simulink model "EV"  (R2022b)
settings: Solver=VariableStepAuto  StartTime=0.0  StopTime=500  RelTol=1e-3
libraries: autolibshared x1, slpidlib x1
settings Model: Creator=frz  LastModifiedBy=frz
settings SolverCC: ZeroCrossAlgorithm=Adaptive
settings DataIOCC: SaveOutput=off  SaveTime=off  ReturnWorkspaceOutputs=off
settings DebuggingCC: IgnoredZcDiagnostic=none

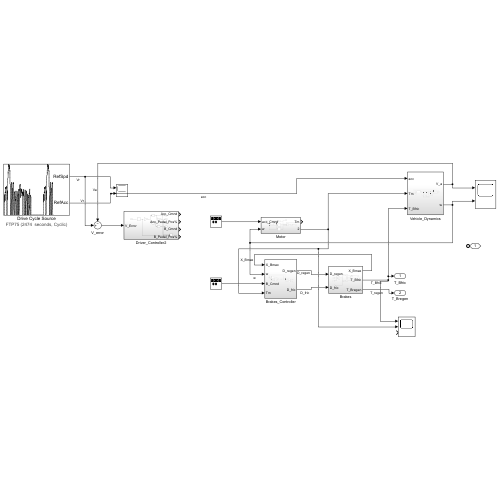
[thumbnail: Simulink's stored preview of the top-level diagram]
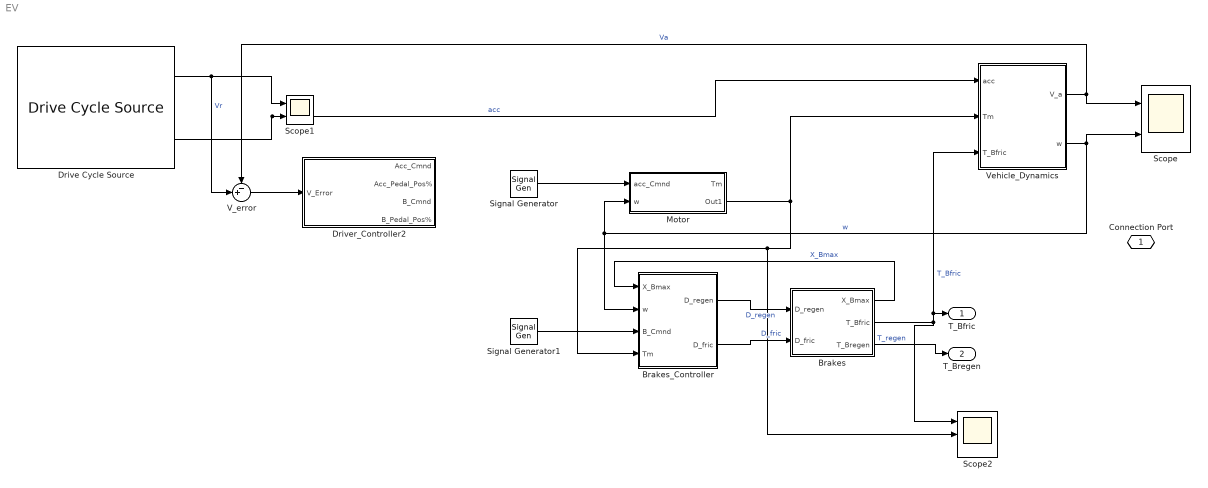
== system EV ==
  Brakes : Subsystem
  Brakes_Controller : Subsystem
  Drive Cycle Source : autolibshared/Drive Cycle Source  cycleVar=FTP75  fileVar=cycleFTP75.mat  tfinal="2474  seconds, Cyclic"  cycleRepeat=on  outAccPort=on  outGearPort=off  gearList=No gear data  t_wot1=5  xdot_woto=0  xdot_wot1=30  t_wot2=20  xdot_wot2=0  t_wotend=30  srcUnit=m/s  outUnit=km/h  srcAccUnit=m/s/s  outAccUnit=km/h^2  dt=0  aMode=1  faultOption=off  velBnd=2  velBndUnit=mph  inUnit=m/s  timeBnd=1  failOption=off  stopSim=off  maxFaultCnt=10  maxFaultTime=2  maxTotFaultTime=15  traceOption=off  dtTrace=1  traceWindow=10  lastDCname=FTP75  lastOutUnit=mph  lastDT=0  lastTB=1  lastSB=2  forceCalcBound=off
  Driver_Controller2 : Subsystem
  Motor : Subsystem
  Scope : Scope  NumInputPorts=2
  Scope1 : Scope  NumInputPorts=2
  Scope2 : Scope  NumInputPorts=3
  Signal Generator : SignalGenerator  Frequency=0.005  Units=rad/sec
  Signal Generator1 : SignalGenerator  Amplitude=-1  Frequency=0.005  Units=rad/sec
  V_error : Sum  Inputs=-+|
  Vehicle_Dynamics : Subsystem
  Connection Port : PMIOPort  Side=Left
  T_Bfric : Outport
  T_Bregen : Outport  Port=2
  wires:
  Drive Cycle Source/1 -> Scope1/1, V_error/2  "Vr"
  Drive Cycle Source/2 -> Scope1/2, Vehicle_Dynamics/1(acc)  "acc"
  Brakes/2(T_Bfric) -> Scope2/1, Vehicle_Dynamics/3(T_Bfric), T_Bfric/1  "T_Bfric"
  Brakes/1(X_Bmax) -> Brakes_Controller/1(X_Bmax)  "X_Bmax"
  Brakes_Controller/1(D_regen) -> Brakes/1(D_regen)  "D_regen"
  Brakes_Controller/2(D_fric) -> Brakes/2(D_fric)  "D_fric"
  Brakes/3(T_Bregen) -> T_Bregen/1  "T_regen"
  Vehicle_Dynamics/2(w) -> Scope/2, Motor/2(w), Brakes_Controller/2(w)  "w"
  Vehicle_Dynamics/1(V_a) -> V_error/1, Scope/1  "Va"
  Motor/2(Out1) -> Vehicle_Dynamics/2(Tm), Scope2/2, Brakes_Controller/4(Tm)
  V_error/1 -> Driver_Controller2/1(V_Error)
  Signal Generator1/1 -> Brakes_Controller/3(B_Cmnd)
  Signal Generator/1 -> Motor/1(acc_Cmnd)

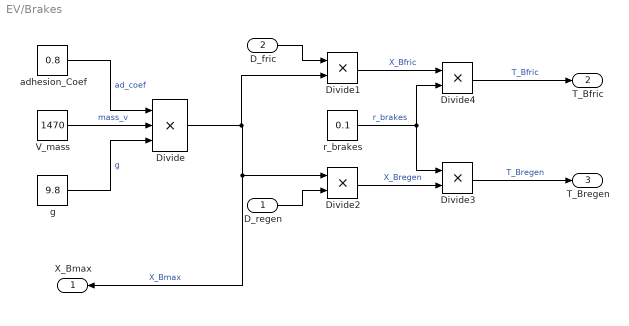
== system EV/Brakes ==
  D_regen : Inport
  D_fric : Inport  Port=2
  Divide : Product  Inputs=***
  Divide{1..4} (4 alike) : Product  Inputs=**
  V_mass : Constant  Value=1470
  adhesion_Coef : Constant  Value=0.8
  g : Constant  Value=9.8
  r_brakes : Constant  Value=0.1
  X_Bmax : Outport
  T_Bfric : Outport  Port=2
  T_Bregen : Outport  Port=3
  wires:
  g/1 -> Divide/3  "g"
  adhesion_Coef/1 -> Divide/1  "ad_coef"
  V_mass/1 -> Divide/2  "mass_v"
  D_fric/1 -> Divide1/1
  Divide1/1 -> Divide4/1  "X_Bfric"
  Divide4/1 -> T_Bfric/1  "T_Bfric"
  r_brakes/1 -> Divide3/1, Divide4/2  "r_brakes"
  D_regen/1 -> Divide2/2
  Divide/1 -> Divide1/2, X_Bmax/1, Divide2/1  "X_Bmax"
  Divide2/1 -> Divide3/2  "X_Bregen"
  Divide3/1 -> T_Bregen/1  "T_Bregen"

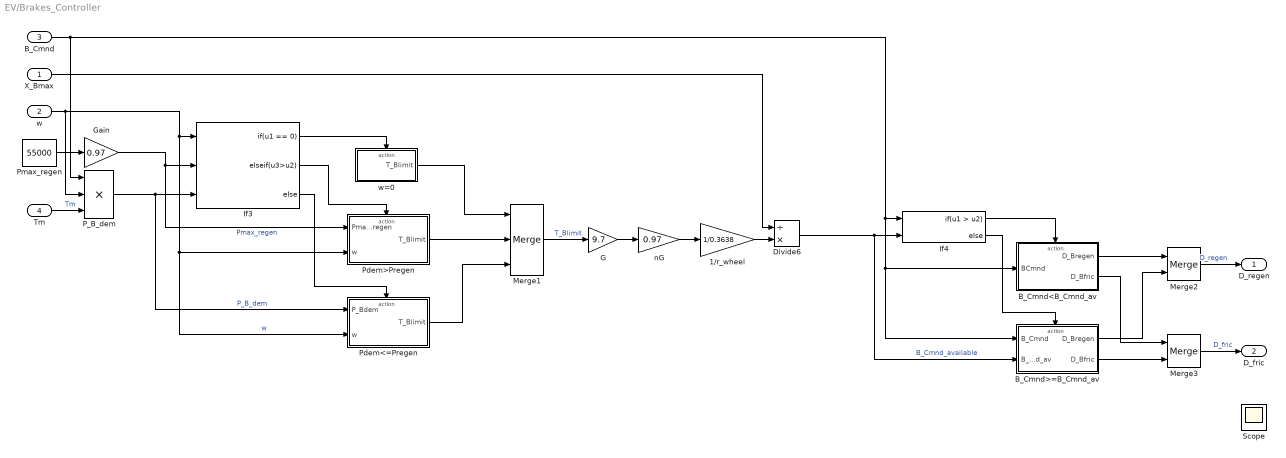
== system EV/Brakes_Controller ==
  X_Bmax : Inport
  w : Inport  Port=2
  B_Cmnd : Inport  Port=3
  Tm : Inport  Port=4
  1/r_wheel : Gain  Gain=1/0.3638
  B_Cmnd<B_Cmnd_av : Subsystem  TreatAsAtomicUnit=on
  B_Cmnd>=B_Cmnd_av : Subsystem  TreatAsAtomicUnit=on
  Divide6 : Product  Inputs=/*
  G : Gain  Gain=9.7
  Gain : Gain  Gain=0.97
  If3 : If  NumInputs=3  IfExpression=u1 == 0  ElseIfExpressions=u3>u2
  If4 : If  NumInputs=2  IfExpression=u1 > u2
  Merge1 : Merge  Inputs=3
  Merge2 : Merge
  Merge3 : Merge
  P_B_dem : Product  Inputs=***
  Pdem<=Pregen : Subsystem  TreatAsAtomicUnit=on
  Pdem>Pregen : Subsystem  TreatAsAtomicUnit=on
  Pmax_regen : Constant  Value=55000
  Scope : Scope
  nG : Gain  Gain=0.97
  w=0 : Subsystem  TreatAsAtomicUnit=on
  D_regen : Outport
  D_fric : Outport  Port=2
  wires:
  Pdem<=Pregen/1(T_Blimit) -> Merge1/3
  If3/1 -> w=0/Action
  Pmax_regen/1 -> Gain/1
  B_Cmnd/1 -> If4/1, B_Cmnd<B_Cmnd_av/1(BCmnd), B_Cmnd>=B_Cmnd_av/1(B_Cmnd), P_B_dem/1
  X_Bmax/1 -> Divide6/1
  Merge2/1 -> D_regen/1  "D_regen"
  If3/2 -> Pdem>Pregen/Action
  P_B_dem/1 -> If3/3, Pdem<=Pregen/1(P_Bdem)  "P_B_dem"
  G/1 -> nG/1
  w/1 -> P_B_dem/2, Pdem>Pregen/2(w), Pdem<=Pregen/2(w), If3/1  "w"
  w=0/1(T_Blimit) -> Merge1/1
  Pdem>Pregen/1(T_Blimit) -> Merge1/2
  B_Cmnd>=B_Cmnd_av/2(D_Bfric) -> Merge3/2
  If3/3 -> Pdem<=Pregen/Action
  1/r_wheel/1 -> Divide6/2
  B_Cmnd<B_Cmnd_av/2(D_Bfric) -> Merge3/1
  B_Cmnd>=B_Cmnd_av/1(D_Bregen) -> Merge2/2
  If4/2 -> B_Cmnd>=B_Cmnd_av/Action
  Divide6/1 -> If4/2, B_Cmnd>=B_Cmnd_av/2(B_Cmnd_av)  "B_Cmnd_available"
  If4/1 -> B_Cmnd<B_Cmnd_av/Action
  nG/1 -> 1/r_wheel/1
  Merge1/1 -> G/1  "T_Blimit"
  B_Cmnd<B_Cmnd_av/1(D_Bregen) -> Merge2/1
  Merge3/1 -> D_fric/1  "D_fric"
  Gain/1 -> If3/2, Pdem>Pregen/1(Pmax_regen)  "Pmax_regen"
  Tm/1 -> P_B_dem/3  "Tm"

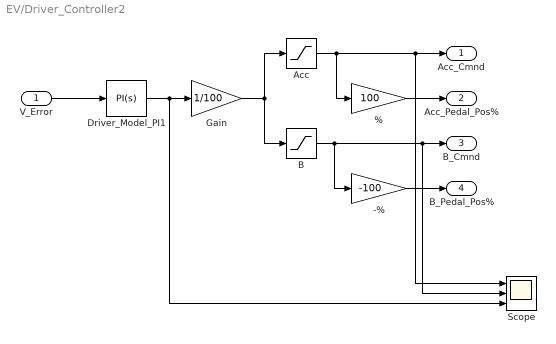
== system EV/Driver_Controller2 ==
  V_Error : Inport
  % : Gain  Gain=100
  -% : Gain  Gain=-100
  Acc : Saturate  UpperLimit=1  LowerLimit=0
  B : Saturate  UpperLimit=0  LowerLimit=-1
  Driver_Model_PI1 : slpidlib/PID Controller  Controller=PI  Form=Parallel  TimeDomain=Continuous-time  UseExternalTs=off  SampleTime=-1  IntegratorMethod=Forward Euler  FilterMethod=Forward Euler  ControllerParametersSource=internal  P=60  I=2  UseKiTs=off  D=0  N=100  UseFilter=on  TunerSelectOption=Transfer Function Based (PID Tuner App)  InitialConditionSource=internal  InitialConditionForIntegrator=0  InitialConditionForFilter=0  DifferentiatorICPrevScaledInput=0  ExternalReset=none  TrackingMode=off  Kt=1  LimitOutput=off  SatLimitsSource=internal  UpperSaturationLimit=inf  LowerSaturationLimit=-inf  LinearizeAsGain=on  AntiWindupMode=none  Kb=1  LimitIntegrator=off  UpperIntegratorSaturationLimit=inf  LowerIntegratorSaturationLimit=-inf  POutMin=[]  POutMax=[]  IOutMin=[]  IOutMax=[]  DOutMin=[]  DOutMax=[]  NOutMin=[]  NOutMax=[]  SumOutMin=[]  SumOutMax=[]  SaturationOutMin=[]  SaturationOutMax=[]  PParamMin=[]  PParamMax=[]  IParamMin=[]  IParamMax=[]  DParamMin=[]  DParamMax=[]  NParamMin=[]  NParamMax=[]  KbParamMin=[]  KbParamMax=[]  KtParamMin=[]  KtParamMax=[]  KbOutMin=[]  KbOutMax=[]  KtOutMin=[]  KtOutMax=[]  IntegratorOutMin=[]  IntegratorOutMax=[]  FilterOutMin=[]  FilterOutMax=[]  SumI1OutMin=[]  SumI1OutMax=[]  SumI2OutMin=[]  SumI2OutMax=[]  SumI3OutMin=[]  SumI3OutMax=[]  SumI4OutMin=[]  SumI4OutMax=[]  SumDOutMin=[]  SumDOutMax=[]  DifferentiatorOutMin=[]  DifferentiatorOutMax=[]  FilterDiffOutCoefMin=[]  FilterDiffOutCoefMax=[]  ReciprocalOutMin=[]  ReciprocalOutMax=[]  SumDenOutMin=[]  SumDenOutMax=[]  SumNumOutMin=[]  SumNumOutMax=[]  DivideOutMin=[]  DivideOutMax=[]  UdiffTsProdOutMin=[]  UdiffTsProdOutMax=[]  NTsProdOutMin=[]  NTsProdOutMax=[]  UintegralTsProdOutMin=[]  UintegralTsProdOutMax=[]  UngainTsProdOutMin=[]  UngainTsProdOutMax=[]  ClampingZeroOutDataTypeStr=Inherit: Inherit via back propagation  ClampingZeroOutMin=[]  ClampingZeroOutMax=[]  FilterDenConstantOutDataTypeStr=Inherit: Inherit via back propagation  FilterDenConstantOutMin=[]  FilterDenConstantOutMax=[]  PCopyOutDataTypeStr=Inherit: Inherit via back propagation  PCopyOutMin=[]  PCopyOutMax=[]  NCopyOutDataTypeStr=Inherit: Inherit via back propagation  NCopyOutMin=[]  NCopyOutMax=[]  IntegratorContinuousStateAttributes=''  IntegratorStateMustResolveToSignalObject=off  IntegratorRTWStateStorageClass=Auto  FilterContinuousStateAttributes=''  FilterStateMustResolveToSignalObject=off  FilterRTWStateStorageClass=Auto  ParallelPVariant=InternalParameters  IdealPVariant=Disabled  IVariant=InternalParameters  DVariant=Disabled  IntegratorVariant=Continuous  SatVariant=Disabled  AWVariant=Passthrough  PCopyVariant=Disabled  TRVariant=Disabled  FdbkBlocksVariant=Forward  IdealPFdbkVariant=Disabled  SatFdbkVariant=Disabled  DerivativeFilterVariant=Disabled  NVariant=Disabled  NCopyVariant=Disabled_SignalSpec  FilterICVariant=Disabled  IntegratorICVariant=InternalICs  ExternalResetVariant=Disabled  TRSumVariant=Passthrough  SumFdbkVariant=Disabled  SumVariant=Sum_PI  TsampFilterVariant=InternalTs  TsampNgainVariant=Passthrough  TsampIntegralVariant=Passthrough  ExternalSaturationOutDataTypeStr=Inherit: Same as second input
  Gain : Gain  Gain=1/100
  Scope : Scope  NumInputPorts=3
  Acc_Cmnd : Outport
  Acc_Pedal_Pos% : Outport  Port=2
  B_Cmnd : Outport  Port=3
  B_Pedal_Pos% : Outport  Port=4
  wires:
  %/1 -> Acc_Pedal_Pos%/1
  -%/1 -> B_Pedal_Pos%/1
  B/1 -> B_Cmnd/1, Scope/2, -%/1
  Acc/1 -> Acc_Cmnd/1, Scope/1, %/1
  V_Error/1 -> Driver_Model_PI1/1
  Driver_Model_PI1/1 -> Scope/3, Gain/1
  Gain/1 -> B/1, Acc/1

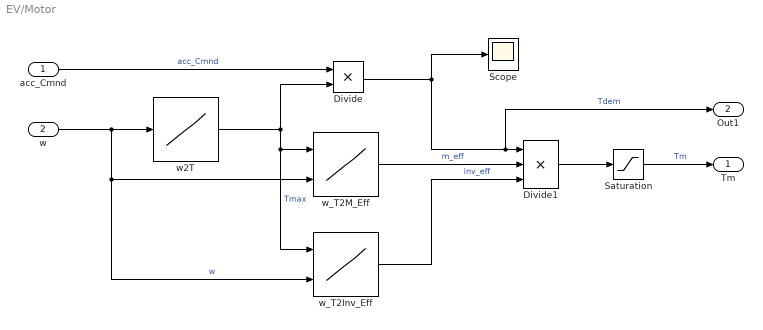
== system EV/Motor ==
  acc_Cmnd : Inport
  w : Inport  Port=2
  Divide : Product  Inputs=**
  Divide1 : Product  Inputs=***
  Saturation : Saturate  UpperLimit=250  LowerLimit=-250
  Scope : Scope
  w2T : Lookup_n-D  NumberOfTableDimensions=1  BreakpointsForDimension1=[0;4700;11400]  Table=[250;250;89]  InternalRulePriority=Speed  RndMeth=Simplest
  w_T2Inv_Eff : Lookup_n-D  BreakpointsForDimension1=[1:3]  BreakpointsForDimension2=[1:3]  InternalRulePriority=Speed  RndMeth=Simplest
      settings: InputPortMap=u0,u1
  w_T2M_Eff : Lookup_n-D  BreakpointsForDimension1=[1:3]  BreakpointsForDimension2=[1:3]  InternalRulePriority=Speed  RndMeth=Simplest
      settings: InputPortMap=u0,u1
  Tm : Outport
  Out1 : Outport  Port=2
  wires:
  w_T2M_Eff/1 -> Divide1/2  "m_eff"
  w2T/1 -> Divide/2, w_T2Inv_Eff/1, w_T2M_Eff/1  "Tmax"
  w/1 -> w2T/1, w_T2Inv_Eff/2, w_T2M_Eff/2  "w"
  Divide/1 -> Scope/1, Out1/1, Divide1/1  "Tdem"
  Saturation/1 -> Tm/1  "Tm"
  w_T2Inv_Eff/1 -> Divide1/3  "inv_eff"
  acc_Cmnd/1 -> Divide/1  "acc_Cmnd"
  Divide1/1 -> Saturation/1

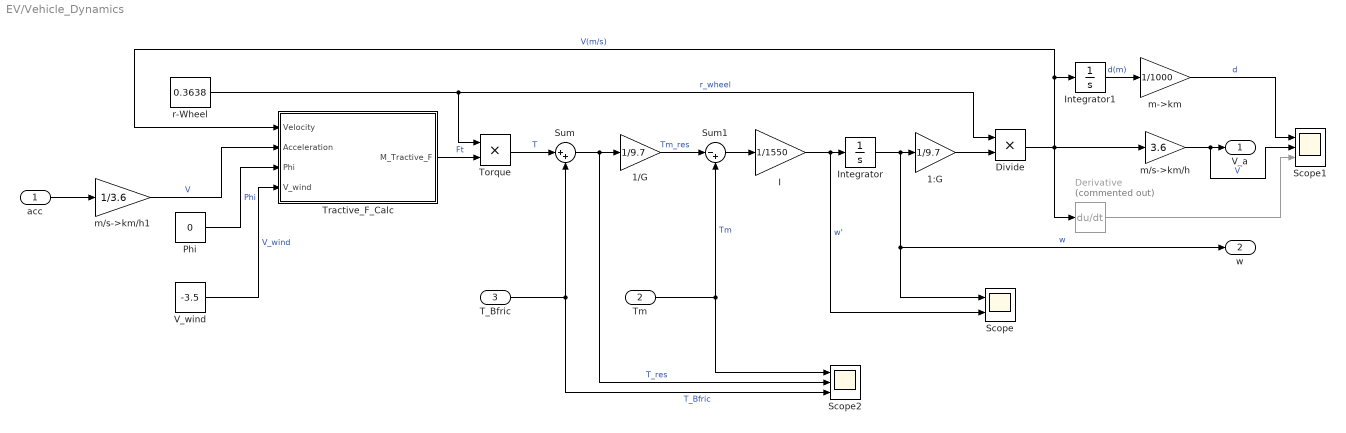
== system EV/Vehicle_Dynamics ==
  acc : Inport
  Tm : Inport  Port=2
  T_Bfric : Inport  Port=3
  1/G : Gain  Gain=1/9.7
  1:G : Gain  Gain=1/9.7
  Derivative : Derivative  Commented=on
  Divide : Product  Inputs=**
  I : Gain  Gain=1/1550
  Integrator : Integrator  LimitOutput=on  UpperSaturationLimit=11400*2*pi/60  LowerSaturationLimit=-11400*2*pi/60
  Integrator1 : Integrator
  Phi : Constant  Value=0
  Scope : Scope  NumInputPorts=2
  Scope1 : Scope  NumInputPorts=3
  Scope2 : Scope  NumInputPorts=3
  Sum : Sum  Inputs=|++
  Sum1 : Sum  Inputs=|-+
  Torque : Product  Inputs=**
  Tractive_F_Calc : Subsystem
  V_wind : Constant  Value=-3.5
  m->km : Gain  Gain=1/1000
  m/s->km/h : Gain  Gain=3.6
  m/s->km/h1 : Gain  Gain=1/3.6
  r-Wheel : Constant  Value=0.3638
  V_a : Outport
  w : Outport  Port=2
  wires:
  m->km/1 -> Scope1/1  "d"
  Sum1/1 -> I/1
  Divide/1 -> Tractive_F_Calc/1(Velocity), Integrator1/1, Derivative/1, m/s->km/h/1  "V(m/s)"
  1:G/1 -> Divide/2
  r-Wheel/1 -> Divide/1, Torque/1  "r_wheel"
  acc/1 -> m/s->km/h1/1
  Integrator1/1 -> m->km/1  "d(m)"
  Torque/1 -> Sum/1  "T"
  Integrator/1 -> Scope/1, w/1, 1:G/1  "w"
  Sum/1 -> Scope2/2, 1/G/1  "T_res"
  V_wind/1 -> Tractive_F_Calc/4(V_wind)  "V_wind"
  I/1 -> Scope/2, Integrator/1  "w'"
  T_Bfric/1 -> Scope2/3, Sum/2  "T_Bfric"
  Tractive_F_Calc/1(M_Tractive_F) -> Torque/2  "Ft"
  Phi/1 -> Tractive_F_Calc/3(Phi)  "Phi"
  Tm/1 -> Scope2/1, Sum1/2  "Tm"
  1/G/1 -> Sum1/1  "Tm_res"
  m/s->km/h/1 -> Scope1/2, V_a/1  "V"
  m/s->km/h1/1 -> Tractive_F_Calc/2(Acceleration)  "V"
  Derivative/1 -> Scope1/3

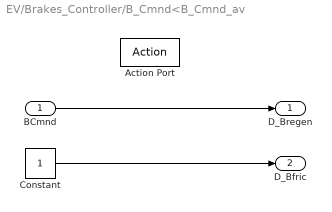
== system EV/Brakes_Controller/B_Cmnd<B_Cmnd_av ==
  BCmnd : Inport
  Action Port : ActionPort  ActionPortLabel=if(u1 > u2)
  Constant : Constant
  D_Bregen : Outport
  D_Bfric : Outport  Port=2
  wires:
  BCmnd/1 -> D_Bregen/1
  Constant/1 -> D_Bfric/1

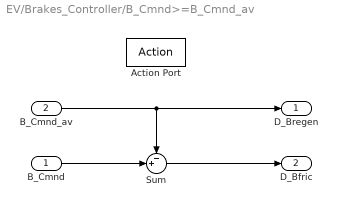
== system EV/Brakes_Controller/B_Cmnd>=B_Cmnd_av ==
  B_Cmnd : Inport
  B_Cmnd_av : Inport  Port=2
  Action Port : ActionPort  ActionPortLabel=else
  Sum : Sum  Inputs=-+|
  D_Bregen : Outport
  D_Bfric : Outport  Port=2
  wires:
  B_Cmnd_av/1 -> Sum/1, D_Bregen/1
  B_Cmnd/1 -> Sum/2
  Sum/1 -> D_Bfric/1

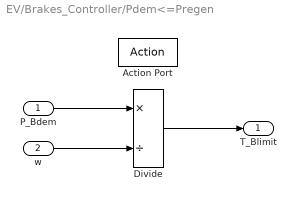
== system EV/Brakes_Controller/Pdem<=Pregen ==
  P_Bdem : Inport
  w : Inport  Port=2
  Action Port : ActionPort  ActionPortLabel=else
  Divide : Product  Inputs=*/
  T_Blimit : Outport
  wires:
  P_Bdem/1 -> Divide/1
  w/1 -> Divide/2
  Divide/1 -> T_Blimit/1

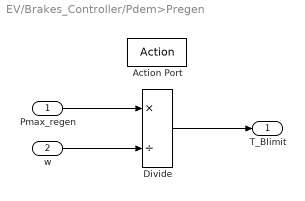
== system EV/Brakes_Controller/Pdem>Pregen ==
  Pmax_regen : Inport
  w : Inport  Port=2
  Action Port : ActionPort  ActionPortLabel=elseif(u3>u2)
  Divide : Product  Inputs=*/
  T_Blimit : Outport
  wires:
  Pmax_regen/1 -> Divide/1
  w/1 -> Divide/2
  Divide/1 -> T_Blimit/1

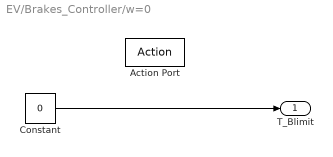
== system EV/Brakes_Controller/w=0 ==
  Action Port : ActionPort  ActionPortLabel=if(u1 == 0)
  Constant : Constant  Value=0
  T_Blimit : Outport
  wires:
  Constant/1 -> T_Blimit/1

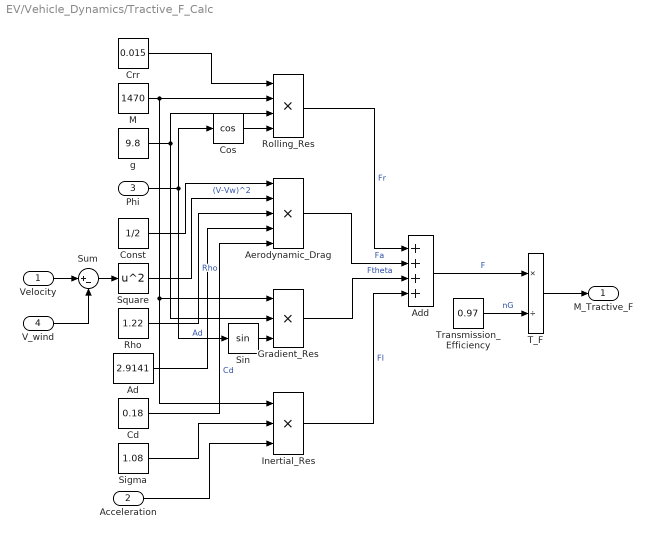
== system EV/Vehicle_Dynamics/Tractive_F_Calc ==
  Velocity : Inport
  Acceleration : Inport  Port=2
  Phi : Inport  Port=3
  V_wind : Inport  Port=4
  Ad : Constant  Value=2.9141
  Add : Sum  Inputs=++++
  Aerodynamic_Drag : Product  Inputs=*****
  Cd : Constant  Value=0.18
  Const : Constant  Value=1/2
  Cos : Trigonometry  Operator=cos
  Crr : Constant  Value=0.015
  Gradient_Res : Product  Inputs=***
  Inertial_Res : Product  Inputs=***
  M : Constant  Value=1470
  Rho : Constant  Value=1.22
  Rolling_Res : Product  Inputs=****
  Sigma : Constant  Value=1.08
  Sin : Trigonometry
  Square : Math  Operator=square
  Sum : Sum  Inputs=|+-
  T_F : Product  Inputs=*/
  Transmission_Efficiency : Constant  Value=0.97
  g : Constant  Value=9.8
  M_Tractive_F : Outport
  wires:
  Rolling_Res/1 -> Add/1  "Fr"
  Sin/1 -> Gradient_Res/3
  Cd/1 -> Aerodynamic_Drag/5  "Cd"
  Add/1 -> T_F/1  "F"
  Inertial_Res/1 -> Add/4  "FI"
  Aerodynamic_Drag/1 -> Add/2  "Fa"
  M/1 -> Inertial_Res/1, Gradient_Res/1, Rolling_Res/2
  Crr/1 -> Rolling_Res/1
  Sigma/1 -> Inertial_Res/2
  Acceleration/1 -> Inertial_Res/3
  g/1 -> Gradient_Res/2, Rolling_Res/3
  Cos/1 -> Rolling_Res/4
  Sum/1 -> Square/1
  Gradient_Res/1 -> Add/3  "Ftheta"
  T_F/1 -> M_Tractive_F/1
  Velocity/1 -> Sum/1
  Ad/1 -> Aerodynamic_Drag/4  "Ad"
  Rho/1 -> Aerodynamic_Drag/3  "Rho"
  Const/1 -> Aerodynamic_Drag/1
  Transmission_Efficiency/1 -> T_F/2  "nG"
  Square/1 -> Aerodynamic_Drag/2  "(V-Vw)^2"
  Phi/1 -> Cos/1, Sin/1
  V_wind/1 -> Sum/2
